simulink model "Cartpole_No_Constraints"  (R2022b)
settings: Solver=VariableStepAuto  StartTime=0.0  StopTime=20  FixedStep=0.1  RelTol=1e-3
settings Model: Creator=rohan  LastModifiedBy=rohan

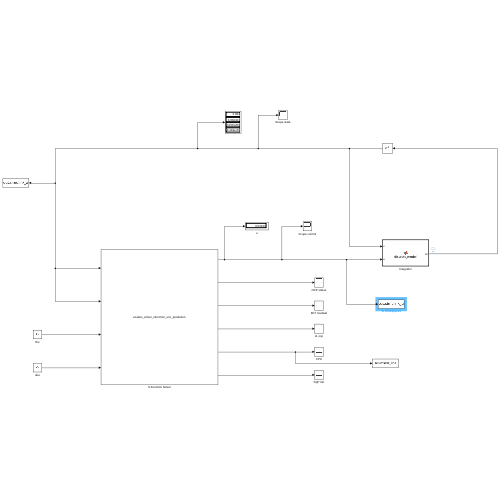
[thumbnail: Simulink's stored preview of the top-level diagram]
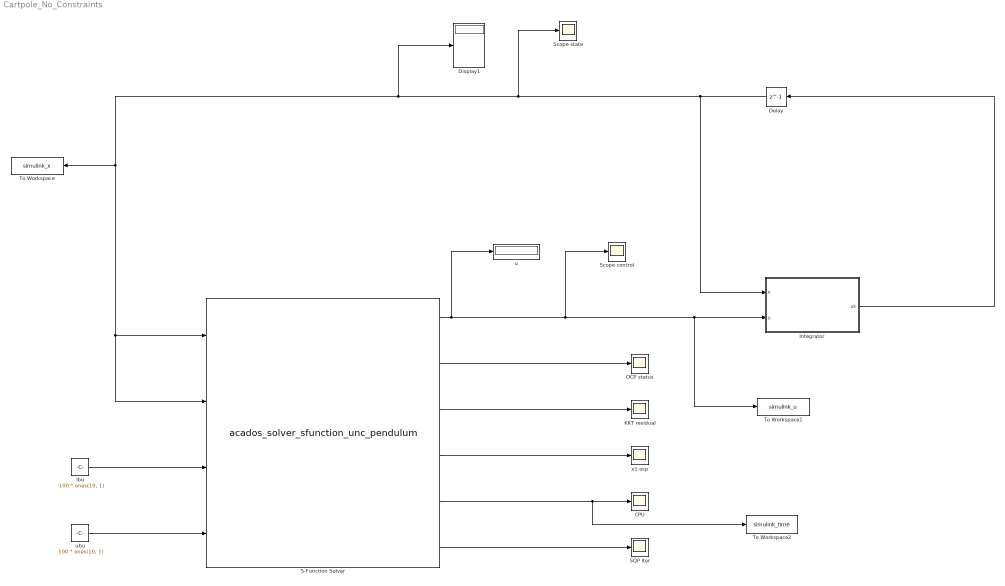
== system Cartpole_No_Constraints ==
  CPU : Scope
      settings: Description=status
  Delay : Delay  DelayLength=1  InitialCondition=[0;0;-pi;0]
  Display1 : Display
  Integrator : MATLAB Function  TreatAsAtomicUnit=on
  KKT residual : Scope
      settings: Description=status
  OCP status : Scope
      settings: Description=status
  S-Function Solver : S-Function  FunctionName=acados_solver_sfunction_unc_pendulum  SFunctionDeploymentMode=off  EnableBusSupport=off
  SQP iter : Scope
      settings: Description=status
  Scope control : Scope
  Scope state : Scope
  To Workspace : ToWorkspace  VariableName=simulink_x  SampleTime=-1
  To Workspace1 : ToWorkspace  VariableName=simulink_u  SampleTime=-1
  To Workspace2 : ToWorkspace  VariableName=simulink_time  SampleTime=-1
  lbu : Constant  Value=-100 * ones(10, 1)
  u : Display
  ubu : Constant  Value=100 * ones(10, 1)
  x1 ocp : Scope
      settings: Description=status
  wires:
  S-Function Solver/6 -> SQP iter/1
  S-Function Solver/5 -> To Workspace2/1, CPU/1
  S-Function Solver/4 -> x1 ocp/1
  S-Function Solver/3 -> KKT residual/1
  S-Function Solver/2 -> OCP status/1
  S-Function Solver/1 -> u/1, To Workspace1/1, Integrator/2(u), Scope control/1
  Integrator/1(xk) -> Delay/1
  Delay/1 -> Integrator/1(x), Scope state/1, Display1/1, To Workspace/1, S-Function Solver/1, S-Function Solver/2
  ubu/1 -> S-Function Solver/4
  lbu/1 -> S-Function Solver/3

== matlab function Cartpole_No_Constraints/Integrator ==
  data: x input; xk output; u input
function xk = discrete_model(x,u)

mCart = 1;  % cart mass
mPend = 1;  % pendulum mass
g = 9.81;   % gravity of earth
L = 0.5;    % pendulum length
Kd = 10;    % cart damping
dt = 0.1;

f = @(x,u) [x(2);...
    (u - Kd*x(2) - mPend*L*x(4)^2*sin(x(3)) + mPend*g*sin(x(3))*cos(x(3))) / (mCart + mPend*sin(x(3))^2);...
    x(4);...
    ((u - Kd*x(2) - mPend*L*x(4)^2*sin(x(3)))*cos(x(3))/(mCart + mPend) + g*sin(x(3))) / (L - mPend*L*cos(x(3))^2/(mCart + mPend))];

for k=1:1 % loop over control intervals
   % Runge-Kutta 4 integration
   k1 = f(x(:,k),         u(:,k));
   k2 = f(x(:,k)+dt/2*k1, u(:,k));
   k3 = f(x(:,k)+dt/2*k2, u(:,k));
   k4 = f(x(:,k)+dt*k3,   u(:,k));
   x_next = x(:,k) + dt/6*(k1+2*k2+2*k3+k4);
end

xk = x_next;

end

function dxdt = Continuous_model(x, u)
 mCart = 1;  % cart mass
 mPend = 1;  % pendulum mass
 g = 9.81;   % gravity of earth
 L = 0.5;    % pendulum length
 Kd = 10;    % cart damping
 %% Obtain x, u and y
 % x
 z_dot = x(2);
 theta = x(3);
 theta_dot = x(4);
 % u
 F = u;
 %% Compute dxdt
 dxdt = x;
 % z_dot
 dxdt(1) = z_dot;
 % z_dot_dot
 dxdt(2) = (F - Kd*z_dot - mPend*L*theta_dot^2*sin(theta) + mPend*g*sin(theta)*cos(theta)) / (mCart + mPend*sin(theta)^2);
 % theta_dot
 dxdt(3) = theta_dot;
 % theta_dot_dot
 dxdt(4) = ((F - Kd*z_dot - mPend*L*theta_dot^2*sin(theta))*cos(theta)/(mCart + mPend) + g*sin(theta)) / (L - mPend*L*cos(theta)^2/(mCart + mPend));
end
